simulink model "AutonomousControl"  (R2015a)
settings: Solver=ode45  StartTime=0.0  StopTime=inf  FixedStep=0.01  RelTol=1e-3
libraries: simulink x11, dspindex x8, dspnetwork x3, aerolibconvert2 x1, IMU_Library x1, GPS_Library x1, realtime_pacer_lib x1, etargetslib x1
(part 1 of 2)
settings Model: xpc_rtwmakecfg_data=_xpcnblib__xpcetherlib__xpcether8255xlib__xpcetherGbElib__xpciplib_  ParamWorkspaceSource=ReferencedWorkspace  CovSFcnEnable=off  Creator=abdkadma  LastModifiedBy=theth
settings OptimizationCC: InlineParams=on  InlineInvariantSignals=on  EnhancedBackFolding=on  ExpressionDepthLimit=2147483647  EfficientFloat2IntCast=on  SimCompilerOptimization=on
settings DebuggingCC: UnderspecifiedInitializationDetection=Classic  MergeDetectMultiDrivingBlocksExec=none  SolverPrmCheckMsg=warning  StateNameClashWarn=warning
settings RTWCC: RTWCompilerOptimization=on  CheckMdlBeforeBuild=Warning
settings GRTTargetCC: MatFileLogging=off  SupportNonFinite=off

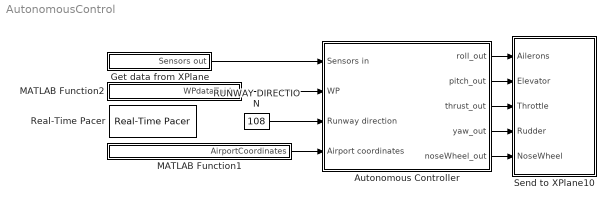
== system AutonomousControl ==
  "Autonomous Controller " : Subsystem
  Get data from XPlane : Subsystem  Description=|  TreatAsAtomicUnit=on  mask(Get Data from Xplane10){remoteURL='127.0.0.1', localPort=49005, sampletime=0.02}
      | Done by: Mohamed Abdelkader
      | Contact for updates: mohamedashraf123@gmail.com
      mask prompts: remoteURL "Remote IP address ('0.0.0.0' to accept all):(default='127.0.0.1')"; localPort "Local IP port: that Xplane10 sends to (default=49005)"; sampletime "Sampling time (seconds), how frequenlty to capture data from Xplane. Don't set to low as it might not be able to capture the smaples from Xplane. Default is 0.02 assuming the UDP rate in Xplane is set to 50 sample per second"
      mask help:
      | Get Data from X-Plane10
      | * make sure you configure the right port
      | and the right IP address
      mask TypeOptions remoteURL: UDP Receive1/remoteURL
      mask TypeOptions localPort: UDP Receive1/localPort
      mask TypeOptions sampletime: UDP Receive1/sampletime
  MATLAB Function1 : MATLAB Function  TreatAsAtomicUnit=on
  MATLAB Function2 : MATLAB Function  TreatAsAtomicUnit=on
  RUNWAY DIRECTION : Constant  Value=108
  Real-Time Pacer : realtime_pacer_lib/Real-Time Pacer  simTimePerRealTime=1
  Send to XPlane10 : Subsystem  Description=|  mask(Send Commands to X-Plane 10){remoteURL='127.0.0.1', remotePort=49000}
      | Done by: Mohamed Abdelkader
      | Contact for updates: mohamedashraf123@gmail.com
      mask prompts: remoteURL "Remote IP address (default='127.0.0.1'): X-Plane10 IP"; remotePort "Remote IP port:X-Plane10 port(default=49000)"
      mask help:
      | Sends Control Surfaces Commands to Xplane10
      | Throttle in [0,1]
      | Elevator, Ailerons, rudder, nosewheel in [-1,1]
      mask TypeOptions remoteURL: UDP Send/remoteURL
      mask TypeOptions remotePort: UDP Send/remotePort
  wires:
  "Autonomous Controller "/1(roll_out) -> Send to XPlane10/1(Ailerons)
  "Autonomous Controller "/2(pitch_out) -> Send to XPlane10/2(Elevator)
  "Autonomous Controller "/3(thrust_out) -> Send to XPlane10/3(Throttle)
  "Autonomous Controller "/4(yaw_out) -> Send to XPlane10/4(Rudder)
  "Autonomous Controller "/5(noseWheel_out) -> Send to XPlane10/5(NoseWheel)
  Get data from XPlane/1(Sensors out) -> "Autonomous Controller "/1(Sensors in)
  RUNWAY DIRECTION/1 -> "Autonomous Controller "/3(Runway direction)
  MATLAB Function1/1(AirportCoordinates) -> "Autonomous Controller "/4(Airport coordinates)
  MATLAB Function2/1(WPdataTable) -> "Autonomous Controller "/2(WP)

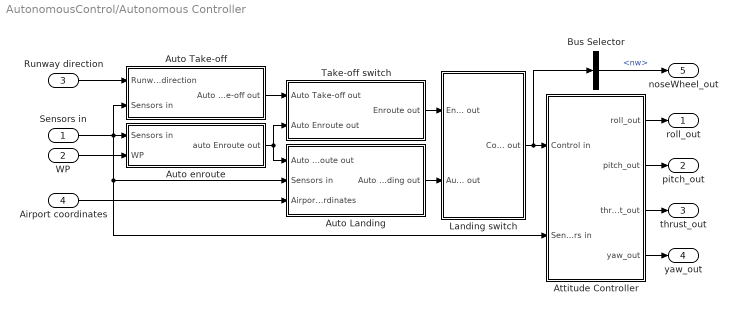
== system AutonomousControl/Autonomous Controller  ==
  Sensors in : Inport
  WP : Inport  Port=2
  Runway direction : Inport  Port=3
  Airport coordinates : Inport  Port=4
  Attitude Controller : Subsystem
  Auto Landing : Subsystem
  Auto Take-off : Subsystem
  Auto enroute : Subsystem
  Bus Selector : BusSelector  OutputSignals=nw
  Landing switch : Subsystem
  Take-off switch : Subsystem
  roll_out : Outport
  pitch_out : Outport  Port=2
  thrust_out : Outport  Port=3
  yaw_out : Outport  Port=4
  noseWheel_out : Outport  Port=5
  wires:
  Take-off switch/1(Enroute out) -> Landing switch/1(Enroute out)
  Auto Landing/1(Auto Landing out) -> Landing switch/2(Auto landing out)
  Auto enroute/1(auto Enroute out) -> Take-off switch/2(Auto Enroute out), Auto Landing/1(Auto Enroute out)
  Attitude Controller/4(yaw_out) -> yaw_out/1
  Attitude Controller/1(roll_out) -> roll_out/1
  Attitude Controller/3(thrust_out) -> thrust_out/1
  Auto Take-off/1(Auto Take-off out) -> Take-off switch/1(Auto Take-off out)
  Sensors in/1 -> Auto Take-off/2(Sensors in), Auto Landing/2(Sensors in), Attitude Controller/2(Sensors in), Auto enroute/1(Sensors in)
  Runway direction/1 -> Auto Take-off/1(Runway direction)
  Landing switch/1(Control out) -> Bus Selector/1, Attitude Controller/1(Control in)
  Bus Selector/1 -> noseWheel_out/1  "<nw>"
  Attitude Controller/2(pitch_out) -> pitch_out/1
  Airport coordinates/1 -> Auto Landing/3(Airport coordinates)
  WP/1 -> Auto enroute/2(WP)

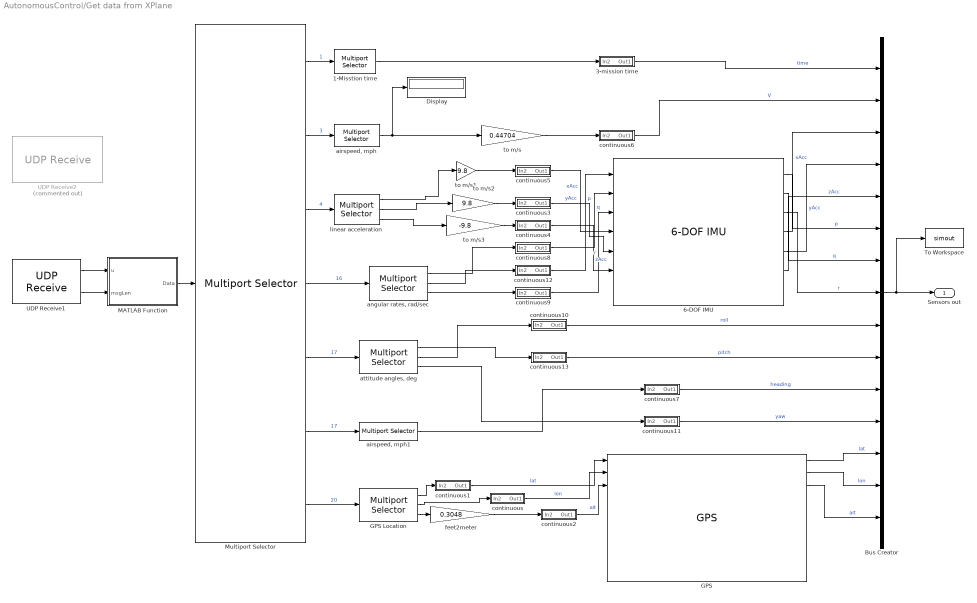
== system AutonomousControl/Get data from XPlane ==
  1-Misstion time : dspindex/Multiport Selector  rowsOrCols=Columns  idxCellArray={3}  idxErrMode=Clip Index
  3-mission time : Subsystem
  6-DOF IMU : IMU_Library/6-DOF IMU  lpf_filt_freq_hz_ix=20 Hz  gyro_scale_ix=+/- 500 deg/sec  accel_scale_ix=+/- 8g  SampleTime=0.02  lpf_filt_freq_hz=5 Hz  gyro_scale=+/- 250 deg/sec  accel_scale=+/- 2g
  Bus Creator : BusCreator  Inputs='time','V','xAcc','yAcc','zAcc','p','q','r','roll','pitch','heading','yaw','lat','lon','alt'
  Display : Display
  GPS : GPS_Library/GPS
  GPS Location : dspindex/Multiport Selector  rowsOrCols=Columns  idxCellArray={1,2,3}  idxErrMode=Clip Index
  MATLAB Function : MATLAB Function  TreatAsAtomicUnit=on
  Multiport Selector : dspindex/Multiport Selector  rowsOrCols=Rows  idxCellArray={1,3,4,16,17,18,20}  idxErrMode=Clip Index
  To Workspace : ToWorkspace  VariableName=simout  SampleTime=-1
      settings: Save2DSignal=2-D array (concatenate along first dimension)
  UDP Receive1 : dspnetwork/UDP Receive  localURL='0.0.0.0'  localPort=localPort  remoteURL=remoteURL  remotePort=-1  recvBufferSize=8192  dims=365*20  signalDatatype=uint8  isVarSize=off  showBlockingTime=off  blockingTime=0  sampletime=sampletime
  UDP Receive2 : dspnetwork/UDP Receive  Commented=on  localURL='0.0.0.0'  localPort=localPort  remoteURL=remoteURL  remotePort=-1  recvBufferSize=8192  dims=365  signalDatatype=uint8  isVarSize=off  showBlockingTime=on  blockingTime=0.01  sampletime=0.01  blockPlatform=LINUX
  "airspeed, mph" : dspindex/Multiport Selector  rowsOrCols=Columns  idxCellArray={6}  idxErrMode=Clip Index
  "airspeed, mph1" : dspindex/Multiport Selector  rowsOrCols=Columns  idxCellArray={3}  idxErrMode=Clip Index
  "angular rates, rad/sec" : dspindex/Multiport Selector  rowsOrCols=Columns  idxCellArray={1,2,3}  idxErrMode=Clip Index
  "attitude angles, deg" : dspindex/Multiport Selector  rowsOrCols=Columns  idxCellArray={1,2,3}  idxErrMode=Clip Index
  continuous : Subsystem
  continuous1 : Subsystem
  continuous10 : Subsystem
  continuous11 : Subsystem
  continuous12 : Subsystem
  continuous13 : Subsystem
  continuous2 : Subsystem
  continuous3 : Subsystem
  continuous4 : Subsystem
  continuous5 : Subsystem
  continuous6 : Subsystem
  continuous7 : Subsystem
  continuous8 : Subsystem
  continuous9 : Subsystem
  feet2meter : Gain  Gain=0.3048
  linear acceleration : dspindex/Multiport Selector  rowsOrCols=Columns  idxCellArray={6,7,5}  idxErrMode=Clip Index
  to m/s : Gain  Gain=0.44704
  to m/s1 : Gain  Gain=9.8
  to m/s2 : Gain  Gain=9.8
  to m/s3 : Gain  Gain=-9.8
  Sensors out : Outport
  wires:
  "attitude angles, deg"/3 -> continuous11/1(In2)
  "angular rates, rad/sec"/3 -> continuous9/1(In2)
  MATLAB Function/1(Data) -> Multiport Selector/1
  linear acceleration/2 -> to m/s2/1
  to m/s2/1 -> continuous3/1(In2)
  to m/s1/1 -> continuous5/1(In2)
  "attitude angles, deg"/1 -> continuous13/1(In2)
  "attitude angles, deg"/2 -> continuous10/1(In2)
  to m/s/1 -> continuous6/1(In2)
  "airspeed, mph"/1 -> Display/1, to m/s/1
  linear acceleration/1 -> to m/s1/1
  "angular rates, rad/sec"/1 -> continuous8/1(In2)
  linear acceleration/3 -> to m/s3/1
  "angular rates, rad/sec"/2 -> continuous12/1(In2)
  "airspeed, mph1"/1 -> continuous7/1(In2)
  to m/s3/1 -> continuous4/1(In2)
  feet2meter/1 -> continuous2/1(In2)
  UDP Receive1/1 -> MATLAB Function/1(u)
  UDP Receive1/2 -> MATLAB Function/2(msgLen)
  GPS Location/3 -> feet2meter/1
  GPS Location/1 -> continuous1/1(In2)
  continuous6/1(Out1) -> Bus Creator/2  "V"
  continuous7/1(Out1) -> Bus Creator/11  "heading"
  continuous10/1(Out1) -> Bus Creator/9  "roll"
  continuous11/1(Out1) -> Bus Creator/12  "yaw"
  continuous13/1(Out1) -> Bus Creator/10  "pitch"
  Bus Creator/1 -> To Workspace/1, Sensors out/1
  Multiport Selector/4 -> "angular rates, rad/sec"/1  "16"
  Multiport Selector/5 -> "attitude angles, deg"/1  "17"
  Multiport Selector/6 -> "airspeed, mph1"/1  "17"
  Multiport Selector/7 -> GPS Location/1  "20"
  1-Misstion time/1 -> 3-mission time/1(In2)
  3-mission time/1(Out1) -> Bus Creator/1  "time"
  Multiport Selector/1 -> 1-Misstion time/1  "1"
  Multiport Selector/2 -> "airspeed, mph"/1  "3"
  Multiport Selector/3 -> linear acceleration/1  "4"
  continuous5/1(Out1) -> 6-DOF IMU/4  "xAcc"
  6-DOF IMU/4 -> Bus Creator/3  "xAcc"
  continuous3/1(Out1) -> 6-DOF IMU/5  "yAcc"
  6-DOF IMU/5 -> Bus Creator/4  "yAcc"
  continuous4/1(Out1) -> 6-DOF IMU/6  "zAcc"
  6-DOF IMU/6 -> Bus Creator/5  "zAcc"
  continuous12/1(Out1) -> 6-DOF IMU/1  "p"
  continuous8/1(Out1) -> 6-DOF IMU/2  "q"
  continuous9/1(Out1) -> 6-DOF IMU/3  "r"
  6-DOF IMU/1 -> Bus Creator/6  "p"
  6-DOF IMU/2 -> Bus Creator/7  "q"
  6-DOF IMU/3 -> Bus Creator/8  "r"
  continuous1/1(Out1) -> GPS/1  "lat"
  GPS/1 -> Bus Creator/13  "lat"
  continuous/1(Out1) -> GPS/2  "lon"
  GPS/2 -> Bus Creator/14  "lon"
  continuous2/1(Out1) -> GPS/3  "alt"
  GPS/3 -> Bus Creator/15  "alt"
  GPS Location/2 -> continuous/1(In2)

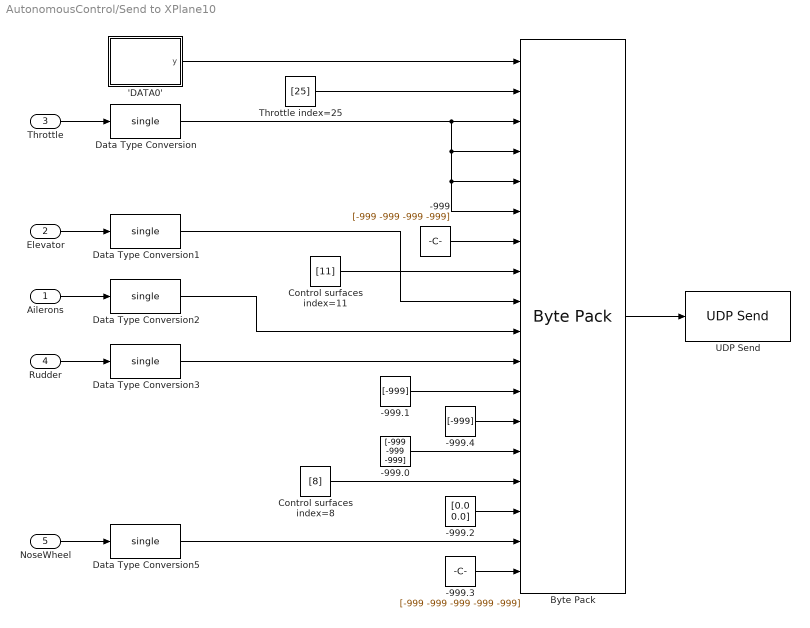
== system AutonomousControl/Send to XPlane10 ==
  Ailerons : Inport
  Elevator : Inport  Port=2
  Throttle : Inport  Port=3
  Rudder : Inport  Port=4
  NoseWheel : Inport  Port=5
  'DATA0' : MATLAB Function  TreatAsAtomicUnit=on
  -999 : Constant  Value=[-999 -999 -999 -999]  OutDataTypeStr=int32  SampleTime=-1
  -999.0 : Constant  Value=[-999 -999 -999]  OutDataTypeStr=int32  SampleTime=-1
  -999.1 : Constant  Value=[-999]  OutDataTypeStr=int32  SampleTime=-1
  -999.2 : Constant  Value=[0.0 0.0]  OutDataTypeStr=single  SampleTime=-1
  -999.3 : Constant  Value=[-999 -999 -999 -999 -999]  OutDataTypeStr=int32  SampleTime=-1
  -999.4 : Constant  Value=[-999]  OutDataTypeStr=single  SampleTime=-1
  Byte Pack : etargetslib/Byte Pack  datatypes={'uint8','uint32','single','single','single','single','int32','uint32','single','single','single','int32','single','int32','uint32','single','single','int32'}  byteAlign=1
  Control surfaces index=11 : Constant  Value=[11]  OutDataTypeStr=uint32  SampleTime=-1
  Control surfaces index=8 : Constant  Value=[8]  OutDataTypeStr=uint32  SampleTime=-1
  Data Type Conversion : DataTypeConversion  OutMin=[0]  OutMax=[1.0]  OutDataTypeStr=single
  Data Type Conversion{1..3,5} (4 alike) : DataTypeConversion  OutMin=[-1.0]  OutMax=[1.0]  OutDataTypeStr=single
  Throttle index=25 : Constant  Value=[25]  OutDataTypeStr=uint32  SampleTime=-1
  UDP Send : dspnetwork/UDP Send  remoteURL=remoteURL  remotePort=remotePort  localURL='0.0.0.0'  localPortSource=Automatically determine  localPort=-1  sampletime=-1  separateLengthPort=0
  wires:
  Ailerons/1 -> Data Type Conversion2/1
  Control surfaces index=11/1 -> Byte Pack/8
  Throttle/1 -> Data Type Conversion/1
  Data Type Conversion1/1 -> Byte Pack/9
  'DATA0'/1(y) -> Byte Pack/1
  Throttle index=25/1 -> Byte Pack/2
  Byte Pack/1 -> UDP Send/1
  -999/1 -> Byte Pack/7
  Data Type Conversion2/1 -> Byte Pack/10
  Data Type Conversion3/1 -> Byte Pack/11
  Rudder/1 -> Data Type Conversion3/1
  -999.0/1 -> Byte Pack/14
  Elevator/1 -> Data Type Conversion1/1
  Data Type Conversion/1 -> Byte Pack/3, Byte Pack/4, Byte Pack/6, Byte Pack/5
  -999.1/1 -> Byte Pack/12
  Control surfaces index=8/1 -> Byte Pack/15
  -999.2/1 -> Byte Pack/16
  Data Type Conversion5/1 -> Byte Pack/17
  NoseWheel/1 -> Data Type Conversion5/1
  -999.3/1 -> Byte Pack/18
  -999.4/1 -> Byte Pack/13

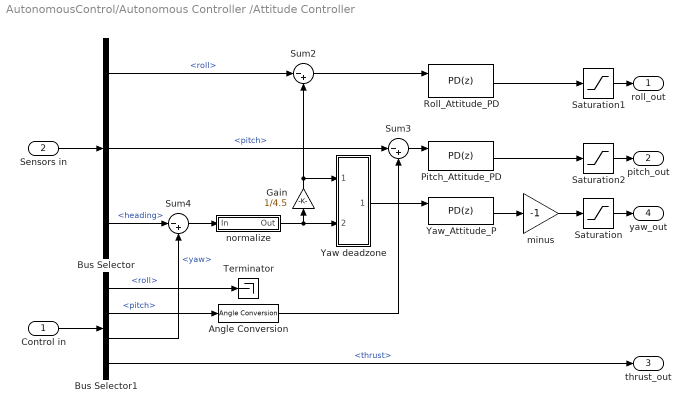
== system AutonomousControl/Autonomous Controller /Attitude Controller ==
  Control in : Inport
  Sensors in : Inport  Port=2
  Angle Conversion : aerolibconvert2/Angle Conversion  IU=rad  OU=deg
  Bus Selector : BusSelector  OutputSignals=roll,pitch,heading
  Bus Selector1 : BusSelector  OutputSignals=roll,pitch,yaw,thrust
  Gain : Gain  Gain=1/4.5
  Pitch_Attitude_PD : simulink/Continuous/PID Controller  Controller=PD  TimeDomain=Discrete-time  SampleTime=0.02  IntegratorMethod=Forward Euler  FilterMethod=Forward Euler  Form=Parallel  UseFilter=off  ControllerParametersSource=internal  P=1*pi/180  I=0  D=0.04*pi/180  N=20  InitialConditionSource=internal  InitialConditionForIntegrator=0  InitialConditionForFilter=0  ExternalReset=either  LimitOutput=on  UpperSaturationLimit=1  LowerSaturationLimit=-1  LinearizeAsGain=on  AntiWindupMode=none  Kb=1  TrackingMode=off  Kt=1  PParamMin=[]  PParamMax=[]  IParamMin=[]  IParamMax=[]  DParamMin=[]  DParamMax=[]  NParamMin=[]  NParamMax=[]  KbParamMin=[]  KbParamMax=[]  KtParamMin=[]  KtParamMax=[]  POutMin=[]  POutMax=[]  IOutMin=[]  IOutMax=[]  DOutMin=[]  DOutMax=[]  NOutMin=[]  NOutMax=[]  KbOutMin=[]  KbOutMax=[]  KtOutMin=[]  KtOutMax=[]  IntegratorOutMin=[]  IntegratorOutMax=[]  FilterOutMin=[]  FilterOutMax=[]  SumOutMin=[]  SumOutMax=[]  SumI1OutMin=[]  SumI1OutMax=[]  SumI2OutMin=[]  SumI2OutMax=[]  SumI3OutMin=[]  SumI3OutMax=[]  SumDOutMin=[]  SumDOutMax=[]  SaturationOutMin=[]  SaturationOutMax=[]  IntegratorContinuousStateAttributes=''  IntegratorStateMustResolveToSignalObject=off  IntegratorRTWStateStorageClass=Auto  FilterContinuousStateAttributes=''  FilterStateMustResolveToSignalObject=off  FilterRTWStateStorageClass=Auto  DifferentiatorICPrevScaledInput=0  DifferentiatorOutMin=[]  DifferentiatorOutMax=[]
  Roll_Attitude_PD : simulink/Continuous/PID Controller  Controller=PD  TimeDomain=Discrete-time  SampleTime=0.02  IntegratorMethod=Forward Euler  FilterMethod=Forward Euler  Form=Parallel  UseFilter=off  ControllerParametersSource=internal  P=pi/180/4  I=0  D=0.0008*pi/180/4  N=20  InitialConditionSource=internal  InitialConditionForIntegrator=0  InitialConditionForFilter=0  ExternalReset=either  LimitOutput=on  UpperSaturationLimit=1  LowerSaturationLimit=-1  LinearizeAsGain=on  AntiWindupMode=none  Kb=1  TrackingMode=off  Kt=1  PParamMin=[]  PParamMax=[]  IParamMin=[]  IParamMax=[]  DParamMin=[]  DParamMax=[]  NParamMin=[]  NParamMax=[]  KbParamMin=[]  KbParamMax=[]  KtParamMin=[]  KtParamMax=[]  POutMin=[]  POutMax=[]  IOutMin=[]  IOutMax=[]  DOutMin=[]  DOutMax=[]  NOutMin=[]  NOutMax=[]  KbOutMin=[]  KbOutMax=[]  KtOutMin=[]  KtOutMax=[]  IntegratorOutMin=[]  IntegratorOutMax=[]  FilterOutMin=[]  FilterOutMax=[]  SumOutMin=[]  SumOutMax=[]  SumI1OutMin=[]  SumI1OutMax=[]  SumI2OutMin=[]  SumI2OutMax=[]  SumI3OutMin=[]  SumI3OutMax=[]  SumDOutMin=[]  SumDOutMax=[]  SaturationOutMin=[]  SaturationOutMax=[]  IntegratorContinuousStateAttributes=''  IntegratorStateMustResolveToSignalObject=off  IntegratorRTWStateStorageClass=Auto  FilterContinuousStateAttributes=''  FilterStateMustResolveToSignalObject=off  FilterRTWStateStorageClass=Auto  DifferentiatorICPrevScaledInput=0  DifferentiatorOutMin=[]  DifferentiatorOutMax=[]
  Saturation : Saturate  UpperLimit=1  LowerLimit=-1
  Saturation1 : Saturate  UpperLimit=0.05  LowerLimit=-0.05
  Saturation2 : Saturate  UpperLimit=1  LowerLimit=-1
  Sum2 : Sum  Inputs=|-+
  Sum3 : Sum  Inputs=|-+
  Sum4 : Sum  Inputs=|-+
  Terminator : Terminator
  Yaw deadzone : Subsystem
  Yaw_Attitude_P : simulink/Continuous/PID Controller  Controller=PD  TimeDomain=Discrete-time  SampleTime=0.02  IntegratorMethod=Forward Euler  FilterMethod=Forward Euler  Form=Parallel  UseFilter=off  ControllerParametersSource=internal  P=6*pi/180  I=0  D=6*0.000034  N=100  InitialConditionSource=internal  InitialConditionForIntegrator=0  InitialConditionForFilter=0  ExternalReset=either  LimitOutput=on  UpperSaturationLimit=1  LowerSaturationLimit=-1  LinearizeAsGain=on  AntiWindupMode=none  Kb=1  TrackingMode=off  Kt=1  PParamMin=[]  PParamMax=[]  IParamMin=[]  IParamMax=[]  DParamMin=[]  DParamMax=[]  NParamMin=[]  NParamMax=[]  KbParamMin=[]  KbParamMax=[]  KtParamMin=[]  KtParamMax=[]  POutMin=[]  POutMax=[]  IOutMin=[]  IOutMax=[]  DOutMin=[]  DOutMax=[]  NOutMin=[]  NOutMax=[]  KbOutMin=[]  KbOutMax=[]  KtOutMin=[]  KtOutMax=[]  IntegratorOutMin=[]  IntegratorOutMax=[]  FilterOutMin=[]  FilterOutMax=[]  SumOutMin=[]  SumOutMax=[]  SumI1OutMin=[]  SumI1OutMax=[]  SumI2OutMin=[]  SumI2OutMax=[]  SumI3OutMin=[]  SumI3OutMax=[]  SumDOutMin=[]  SumDOutMax=[]  SaturationOutMin=[]  SaturationOutMax=[]  IntegratorContinuousStateAttributes=''  IntegratorStateMustResolveToSignalObject=off  IntegratorRTWStateStorageClass=Auto  FilterContinuousStateAttributes=''  FilterStateMustResolveToSignalObject=off  FilterRTWStateStorageClass=Auto  DifferentiatorICPrevScaledInput=0  DifferentiatorOutMin=[]  DifferentiatorOutMax=[]
  minus : Gain  Gain=-1
  normalize : Subsystem
  roll_out : Outport
  pitch_out : Outport  Port=2
  thrust_out : Outport  Port=3
  yaw_out : Outport  Port=4
  wires:
  Sum2/1 -> Roll_Attitude_PD/1
  Sum3/1 -> Pitch_Attitude_PD/1
  Bus Selector/1 -> Sum2/1  "<roll>"
  Bus Selector/2 -> Sum3/1  "<pitch>"
  minus/1 -> Saturation/1
  Bus Selector/3 -> Sum4/1  "<heading>"
  Sum4/1 -> normalize/1(In)
  Sensors in/1 -> Bus Selector/1
  Control in/1 -> Bus Selector1/1
  Bus Selector1/2 -> Angle Conversion/1  "<pitch>"
  Bus Selector1/4 -> thrust_out/1  "<thrust>"
  Bus Selector1/3 -> Sum4/2  "<yaw>"
  Saturation1/1 -> roll_out/1
  Saturation2/1 -> pitch_out/1
  Yaw_Attitude_P/1 -> minus/1
  Pitch_Attitude_PD/1 -> Saturation2/1
  Roll_Attitude_PD/1 -> Saturation1/1
  Saturation/1 -> yaw_out/1
  Gain/1 -> Sum2/2, Yaw deadzone/1(Roll)
  Angle Conversion/1 -> Sum3/2
  normalize/1(Out) -> Gain/1, Yaw deadzone/2(in)
  Yaw deadzone/1(out) -> Yaw_Attitude_P/1
  Bus Selector1/1 -> Terminator/1  "<roll>"

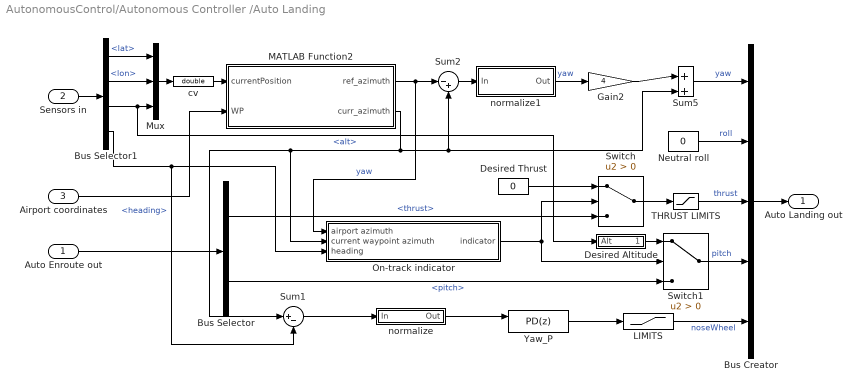
== system AutonomousControl/Autonomous Controller /Auto Landing ==
  Auto Enroute out : Inport
  Sensors in : Inport  Port=2
  Airport coordinates : Inport  Port=3
  Bus Creator : BusCreator  Inputs='yaw','roll','thrust','pitch','noseWheel'
  Bus Selector : BusSelector  OutputSignals=thrust,pitch
  Bus Selector1 : BusSelector  OutputSignals=lat,lon,alt,heading
  Desired Altitude : Subsystem
  Desired Thrust : Constant  Value=0  OutDataTypeStr=single
  Gain2 : Gain  Gain=4
  LIMITS : Saturate
  MATLAB Function2 : MATLAB Function  TreatAsAtomicUnit=on
  Mux : Mux  Inputs=3
  Neutral roll : Constant  Value=0  OutDataTypeStr=single
  On-track indicator : Subsystem
  Sum1 : Sum  Inputs=|+-
  Sum2 : Sum  Inputs=|-+
  Sum5 : Sum  Inputs=|++
  Switch : Switch  Criteria=u2 > Threshold
  Switch1 : Switch  Criteria=u2 > Threshold
  THRUST LIMITS : Saturate  UpperLimit=1  LowerLimit=0
  Yaw_P : simulink/Continuous/PID Controller  Controller=PD  TimeDomain=Discrete-time  SampleTime=0.05  IntegratorMethod=Forward Euler  FilterMethod=Forward Euler  Form=Parallel  UseFilter=off  ControllerParametersSource=internal  P=0.016  I=0  D=0.0024  N=100  InitialConditionSource=internal  InitialConditionForIntegrator=0  InitialConditionForFilter=0  ExternalReset=either  LimitOutput=on  UpperSaturationLimit=1  LowerSaturationLimit=-1  LinearizeAsGain=on  AntiWindupMode=none  Kb=1  TrackingMode=off  Kt=1  PParamMin=[]  PParamMax=[]  IParamMin=[]  IParamMax=[]  DParamMin=[]  DParamMax=[]  NParamMin=[]  NParamMax=[]  KbParamMin=[]  KbParamMax=[]  KtParamMin=[]  KtParamMax=[]  POutMin=[]  POutMax=[]  IOutMin=[]  IOutMax=[]  DOutMin=[]  DOutMax=[]  NOutMin=[]  NOutMax=[]  KbOutMin=[]  KbOutMax=[]  KtOutMin=[]  KtOutMax=[]  IntegratorOutMin=[]  IntegratorOutMax=[]  FilterOutMin=[]  FilterOutMax=[]  SumOutMin=[]  SumOutMax=[]  SumI1OutMin=[]  SumI1OutMax=[]  SumI2OutMin=[]  SumI2OutMax=[]  SumI3OutMin=[]  SumI3OutMax=[]  SumDOutMin=[]  SumDOutMax=[]  SaturationOutMin=[]  SaturationOutMax=[]  IntegratorContinuousStateAttributes=''  IntegratorStateMustResolveToSignalObject=off  IntegratorRTWStateStorageClass=Auto  FilterContinuousStateAttributes=''  FilterStateMustResolveToSignalObject=off  FilterRTWStateStorageClass=Auto  DifferentiatorICPrevScaledInput=0  DifferentiatorOutMin=[]  DifferentiatorOutMax=[]
  cv : DataTypeConversion  OutDataTypeStr=double
  normalize : Subsystem
  normalize1 : Subsystem
  Auto Landing out : Outport
  wires:
  THRUST LIMITS/1 -> Bus Creator/3  "thrust"
  Airport coordinates/1 -> MATLAB Function2/2(WP)
  MATLAB Function2/2(curr_azimuth) -> Sum1/1, On-track indicator/2(current waypoint azimuth), Sum5/2, Sum2/2
  LIMITS/1 -> Bus Creator/5  "noseWheel"
  MATLAB Function2/1(ref_azimuth) -> Sum2/1, On-track indicator/1(airport azimuth)  "yaw"
  normalize/1(Out) -> Yaw_P/1
  Auto Enroute out/1 -> Bus Selector/1
  Bus Selector/1 -> Switch/3  "<thrust>"
  Neutral roll/1 -> Bus Creator/2  "roll"
  Sum1/1 -> normalize/1(In)
  Bus Creator/1 -> Auto Landing out/1
  Sensors in/1 -> Bus Selector1/1
  Bus Selector1/1 -> Mux/1  "<lat>"
  Bus Selector1/2 -> Mux/2  "<lon>"
  Bus Selector1/3 -> Desired Altitude/1(Alt), Mux/3  "<alt>"
  Sum2/1 -> normalize1/1(In)
  Bus Selector1/4 -> Sum1/2, On-track indicator/3(heading)  "<heading>"
  Desired Thrust/1 -> Switch/1
  Bus Selector/2 -> Switch1/3  "<pitch>"
  Switch/1 -> THRUST LIMITS/1
  Switch1/1 -> Bus Creator/4  "pitch"
  normalize1/1(Out) -> Gain2/1  "yaw"
  Sum5/1 -> Bus Creator/1  "yaw"
  On-track indicator/1(indicator) -> Switch1/2, Switch/2
  Gain2/1 -> Sum5/1
  Mux/1 -> cv/1
  cv/1 -> MATLAB Function2/1(currentPosition)
  Yaw_P/1 -> LIMITS/1
  Desired Altitude/1(pitch) -> Switch1/1

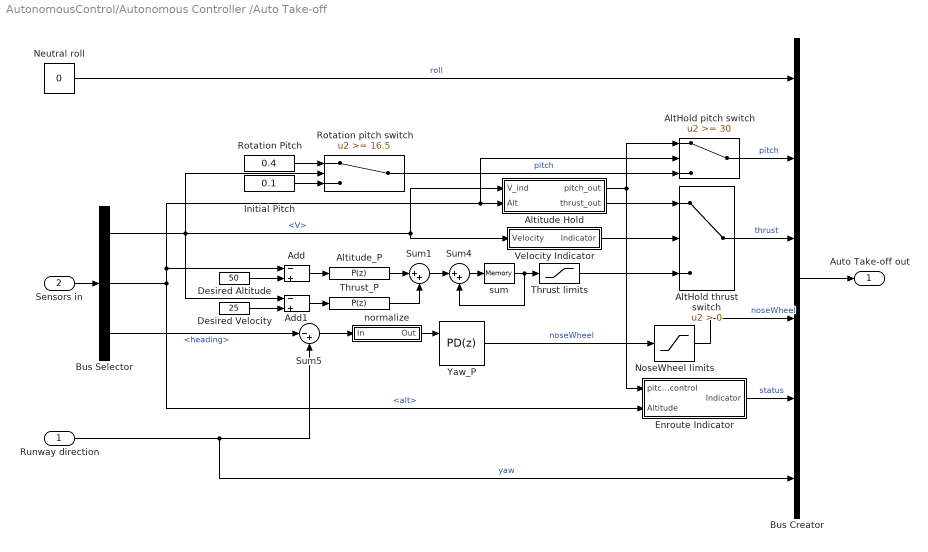
== system AutonomousControl/Autonomous Controller /Auto Take-off ==
  Runway direction : Inport
  Sensors in : Inport  Port=2
  Add : Sum  Inputs=-+
  Add1 : Sum  Inputs=-+
  AltHold pitch switch : Switch  Threshold=30
  AltHold thrust switch : Switch  Criteria=u2 > Threshold
  Altitude Hold : Subsystem
  Altitude_P : simulink/Continuous/PID Controller  Controller=P  TimeDomain=Discrete-time  SampleTime=-1  IntegratorMethod=Forward Euler  FilterMethod=Forward Euler  Form=Parallel  UseFilter=on  ControllerParametersSource=internal  P=0.1  I=0  D=0.01  N=20  InitialConditionSource=internal  InitialConditionForIntegrator=0  InitialConditionForFilter=0  ExternalReset=either  LimitOutput=on  UpperSaturationLimit=1  LowerSaturationLimit=-1  LinearizeAsGain=on  AntiWindupMode=none  Kb=1  TrackingMode=off  Kt=1  PParamMin=[]  PParamMax=[]  IParamMin=[]  IParamMax=[]  DParamMin=[]  DParamMax=[]  NParamMin=[]  NParamMax=[]  KbParamMin=[]  KbParamMax=[]  KtParamMin=[]  KtParamMax=[]  POutMin=[]  POutMax=[]  IOutMin=[]  IOutMax=[]  DOutMin=[]  DOutMax=[]  NOutMin=[]  NOutMax=[]  KbOutMin=[]  KbOutMax=[]  KtOutMin=[]  KtOutMax=[]  IntegratorOutMin=[]  IntegratorOutMax=[]  FilterOutMin=[]  FilterOutMax=[]  SumOutMin=[]  SumOutMax=[]  SumI1OutMin=[]  SumI1OutMax=[]  SumI2OutMin=[]  SumI2OutMax=[]  SumI3OutMin=[]  SumI3OutMax=[]  SumDOutMin=[]  SumDOutMax=[]  SaturationOutMin=[]  SaturationOutMax=[]  IntegratorContinuousStateAttributes=''  IntegratorStateMustResolveToSignalObject=off  IntegratorRTWStateStorageClass=Auto  FilterContinuousStateAttributes=''  FilterStateMustResolveToSignalObject=off  FilterRTWStateStorageClass=Auto  DifferentiatorICPrevScaledInput=0  DifferentiatorOutMin=[]  DifferentiatorOutMax=[]
  Bus Creator : BusCreator  Inputs='roll','pitch','thrust','noseWheel','status','yaw'
  Bus Selector : BusSelector  OutputSignals=V,alt,heading
  Desired Altitude : Constant  Value=50  OutDataTypeStr=single
  Desired Velocity : Constant  Value=25  OutDataTypeStr=single
  Enroute Indicator : Subsystem
  Initial Pitch : Constant  Value=0.1  OutDataTypeStr=single
  Neutral roll : Constant  Value=0  OutDataTypeStr=single
  NoseWheel limits : Saturate
  Rotation Pitch : Constant  Value=0.4  OutDataTypeStr=single
  Rotation pitch switch : Switch  Threshold=16.5
  Sum1 : Sum  Inputs=|++
  Sum4 : Sum  Inputs=|++
  Sum5 : Sum  Inputs=|-+
  Thrust limits : Saturate  UpperLimit=1  LowerLimit=0
  Thrust_P : simulink/Continuous/PID Controller  Controller=P  TimeDomain=Discrete-time  SampleTime=-1  IntegratorMethod=Forward Euler  FilterMethod=Forward Euler  Form=Parallel  UseFilter=on  ControllerParametersSource=internal  P=0.1  I=0  D=0.01  N=20  InitialConditionSource=internal  InitialConditionForIntegrator=0  InitialConditionForFilter=0  ExternalReset=either  LimitOutput=on  UpperSaturationLimit=1  LowerSaturationLimit=-1  LinearizeAsGain=on  AntiWindupMode=none  Kb=1  TrackingMode=off  Kt=1  PParamMin=[]  PParamMax=[]  IParamMin=[]  IParamMax=[]  DParamMin=[]  DParamMax=[]  NParamMin=[]  NParamMax=[]  KbParamMin=[]  KbParamMax=[]  KtParamMin=[]  KtParamMax=[]  POutMin=[]  POutMax=[]  IOutMin=[]  IOutMax=[]  DOutMin=[]  DOutMax=[]  NOutMin=[]  NOutMax=[]  KbOutMin=[]  KbOutMax=[]  KtOutMin=[]  KtOutMax=[]  IntegratorOutMin=[]  IntegratorOutMax=[]  FilterOutMin=[]  FilterOutMax=[]  SumOutMin=[]  SumOutMax=[]  SumI1OutMin=[]  SumI1OutMax=[]  SumI2OutMin=[]  SumI2OutMax=[]  SumI3OutMin=[]  SumI3OutMax=[]  SumDOutMin=[]  SumDOutMax=[]  SaturationOutMin=[]  SaturationOutMax=[]  IntegratorContinuousStateAttributes=''  IntegratorStateMustResolveToSignalObject=off  IntegratorRTWStateStorageClass=Auto  FilterContinuousStateAttributes=''  FilterStateMustResolveToSignalObject=off  FilterRTWStateStorageClass=Auto  DifferentiatorICPrevScaledInput=0  DifferentiatorOutMin=[]  DifferentiatorOutMax=[]
  Velocity Indicator : Subsystem
  Yaw_P : simulink/Continuous/PID Controller  Controller=PD  TimeDomain=Discrete-time  SampleTime=0.02  IntegratorMethod=Forward Euler  FilterMethod=Forward Euler  Form=Parallel  UseFilter=off  ControllerParametersSource=internal  P=0.012  I=0  D=0.0024  N=100  InitialConditionSource=internal  InitialConditionForIntegrator=0  InitialConditionForFilter=0  ExternalReset=either  LimitOutput=on  UpperSaturationLimit=1  LowerSaturationLimit=-1  LinearizeAsGain=on  AntiWindupMode=none  Kb=1  TrackingMode=off  Kt=1  PParamMin=[]  PParamMax=[]  IParamMin=[]  IParamMax=[]  DParamMin=[]  DParamMax=[]  NParamMin=[]  NParamMax=[]  KbParamMin=[]  KbParamMax=[]  KtParamMin=[]  KtParamMax=[]  POutMin=[]  POutMax=[]  IOutMin=[]  IOutMax=[]  DOutMin=[]  DOutMax=[]  NOutMin=[]  NOutMax=[]  KbOutMin=[]  KbOutMax=[]  KtOutMin=[]  KtOutMax=[]  IntegratorOutMin=[]  IntegratorOutMax=[]  FilterOutMin=[]  FilterOutMax=[]  SumOutMin=[]  SumOutMax=[]  SumI1OutMin=[]  SumI1OutMax=[]  SumI2OutMin=[]  SumI2OutMax=[]  SumI3OutMin=[]  SumI3OutMax=[]  SumDOutMin=[]  SumDOutMax=[]  SaturationOutMin=[]  SaturationOutMax=[]  IntegratorContinuousStateAttributes=''  IntegratorStateMustResolveToSignalObject=off  IntegratorRTWStateStorageClass=Auto  FilterContinuousStateAttributes=''  FilterStateMustResolveToSignalObject=off  FilterRTWStateStorageClass=Auto  DifferentiatorICPrevScaledInput=0  DifferentiatorOutMin=[]  DifferentiatorOutMax=[]
  normalize : Subsystem
  sum : Memory
  Auto Take-off out : Outport
  wires:
  Rotation Pitch/1 -> Rotation pitch switch/1
  Initial Pitch/1 -> Rotation pitch switch/3
  Neutral roll/1 -> Bus Creator/1  "roll"
  Add1/1 -> Thrust_P/1
  Desired Velocity/1 -> Add1/2
  Altitude_P/1 -> Sum1/1
  Add/1 -> Altitude_P/1
  Desired Altitude/1 -> Add/2
  sum/1 -> Sum4/2, Thrust limits/1
  Sum4/1 -> sum/1
  Bus Selector/3 -> Sum5/1  "<heading>"
  Runway direction/1 -> Sum5/2, Bus Creator/6  "yaw"
  Bus Selector/2 -> AltHold pitch switch/2, Altitude Hold/2(Alt), Add/1, Enroute Indicator/2(Altitude)  "<alt>"
  Bus Selector/1 -> Rotation pitch switch/2, Altitude Hold/1(V_ind), Velocity Indicator/1(Velocity), Add1/1  "<V>"
  Sum5/1 -> normalize/1(In)
  normalize/1(Out) -> Yaw_P/1
  Enroute Indicator/1(Indicator) -> Bus Creator/5  "status"
  Bus Creator/1 -> Auto Take-off out/1
  Sensors in/1 -> Bus Selector/1
  AltHold pitch switch/1 -> Bus Creator/2  "pitch"
  Rotation pitch switch/1 -> AltHold pitch switch/3  "pitch"
  Sum1/1 -> Sum4/1
  Thrust_P/1 -> Sum1/2
  AltHold thrust switch/1 -> Bus Creator/3  "thrust"
  Altitude Hold/2(thrust_out) -> AltHold thrust switch/1
  Altitude Hold/1(pitch_out) -> Enroute Indicator/1(pitch control), AltHold pitch switch/1
  Velocity Indicator/1(Indicator) -> AltHold thrust switch/2
  Yaw_P/1 -> NoseWheel limits/1  "noseWheel"
  Thrust limits/1 -> AltHold thrust switch/3
  NoseWheel limits/1 -> Bus Creator/4  "noseWheel"

== system AutonomousControl/Autonomous Controller /Auto enroute ==
  Sensors in : Inport
  WP : Inport  Port=2
  Altitude Hold : Subsystem
  Bus Creator : BusCreator  Inputs='roll','pitch','thrust','yaw','status'
  Bus Selector : BusSelector  OutputSignals=V,lat,lon,alt
  Data Type Conversion : DataTypeConversion  OutDataTypeStr=double
  MATLAB Function2 : MATLAB Function  TreatAsAtomicUnit=on
  Mux : Mux  Inputs=3
  Neutral Roll : Constant  Value=0
  auto Enroute out : Outport
  wires:
  Bus Selector/1 -> Altitude Hold/1(V_ind)  "<V>"
  WP/1 -> MATLAB Function2/2(WP)
  MATLAB Function2/1(targetHeading) -> Bus Creator/4  "yaw"
  MATLAB Function2/2(status) -> Bus Creator/5  "status"
  Neutral Roll/1 -> Bus Creator/1  "roll"
  Bus Creator/1 -> auto Enroute out/1
  Altitude Hold/1(pitch_out) -> Bus Creator/2  "pitch"
  Altitude Hold/2(thrust_out) -> Bus Creator/3  "thrust"
  Sensors in/1 -> Bus Selector/1
  Bus Selector/2 -> Mux/1  "<lat>"
  Bus Selector/3 -> Mux/2  "<lon>"
  Bus Selector/4 -> Altitude Hold/2(Alt), Mux/3  "<alt>"
  Mux/1 -> Data Type Conversion/1
  Data Type Conversion/1 -> MATLAB Function2/1(currentPosition)

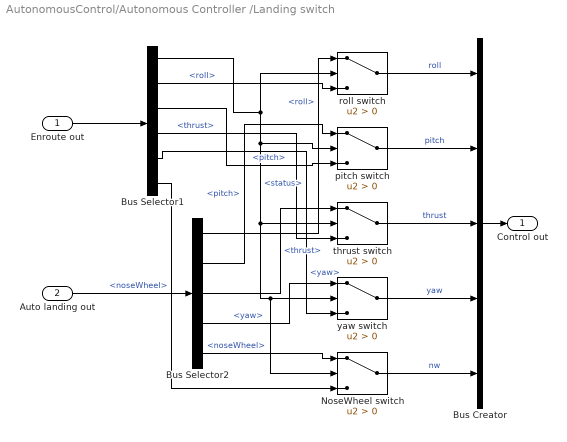
== system AutonomousControl/Autonomous Controller /Landing switch ==
  Enroute out : Inport
  Auto landing out : Inport  Port=2
  Bus Creator : BusCreator  Inputs='roll','pitch','thrust','yaw','nw'
  Bus Selector1 : BusSelector  OutputSignals=status,roll,pitch,thrust,yaw,noseWheel
  Bus Selector2 : BusSelector  OutputSignals=roll,pitch,thrust,yaw,noseWheel
  NoseWheel switch : Switch  Criteria=u2 > Threshold
  pitch switch : Switch  Criteria=u2 > Threshold
  roll switch : Switch  Criteria=u2 > Threshold
  thrust switch : Switch  Criteria=u2 > Threshold
  yaw switch : Switch  Criteria=u2 > Threshold
  Control out : Outport
  wires:
  Bus Selector1/2 -> roll switch/3  "<roll>"
  roll switch/1 -> Bus Creator/1  "roll"
  Bus Selector2/1 -> roll switch/1  "<roll>"
  Bus Selector1/3 -> pitch switch/3  "<pitch>"
  pitch switch/1 -> Bus Creator/2  "pitch"
  Bus Selector2/2 -> pitch switch/1  "<pitch>"
  Bus Selector1/4 -> thrust switch/3  "<thrust>"
  thrust switch/1 -> Bus Creator/3  "thrust"
  Bus Selector2/3 -> thrust switch/1  "<thrust>"
  Bus Selector1/5 -> yaw switch/3  "<yaw>"
  yaw switch/1 -> Bus Creator/4  "yaw"
  Bus Selector2/4 -> yaw switch/1  "<yaw>"
  Bus Selector1/1 -> roll switch/2, NoseWheel switch/2, yaw switch/2, thrust switch/2, pitch switch/2  "<status>"
  Bus Selector1/6 -> NoseWheel switch/3  "<noseWheel>"
  Bus Selector2/5 -> NoseWheel switch/1  "<noseWheel>"
  Enroute out/1 -> Bus Selector1/1
  Auto landing out/1 -> Bus Selector2/1
  Bus Creator/1 -> Control out/1
  NoseWheel switch/1 -> Bus Creator/5  "nw"

== system AutonomousControl/Autonomous Controller /Take-off switch ==
  Auto Take-off out : Inport
  Auto Enroute out : Inport  Port=2
  Bus Creator : BusCreator  Inputs='roll','pitch','thrust','yaw','noseWheel','status'
  Bus Selector : BusSelector  OutputSignals=roll,pitch,thrust,yaw,status
  Bus Selector1 : BusSelector  OutputSignals=status,roll,pitch,thrust,yaw,noseWheel
  pitch switch : Switch  Criteria=u2 > Threshold
  roll switch : Switch  Criteria=u2 > Threshold
  thrust switch : Switch  Criteria=u2 > Threshold
  yaw switch : Switch  Criteria=u2 > Threshold
  Enroute out : Outport
  wires:
  Bus Selector1/2 -> roll switch/3  "<roll>"
  roll switch/1 -> Bus Creator/1  "roll"
  Bus Selector1/3 -> pitch switch/3  "<pitch>"
  pitch switch/1 -> Bus Creator/2  "pitch"
  Bus Selector1/4 -> thrust switch/3  "<thrust>"
  thrust switch/1 -> Bus Creator/3  "thrust"
  Bus Selector1/1 -> yaw switch/2, thrust switch/2, pitch switch/2, roll switch/2  "<status>"
  Bus Selector1/5 -> yaw switch/3  "<yaw>"
  yaw switch/1 -> Bus Creator/4  "yaw"
  Bus Selector/1 -> roll switch/1  "<roll>"
  Bus Selector/2 -> pitch switch/1  "<pitch>"
  Bus Selector/3 -> thrust switch/1  "<thrust>"
  Bus Selector/4 -> yaw switch/1  "<yaw>"
  Auto Enroute out/1 -> Bus Selector/1
  Auto Take-off out/1 -> Bus Selector1/1
  Bus Selector1/6 -> Bus Creator/5  "<noseWheel>"
  Bus Creator/1 -> Enroute out/1
  Bus Selector/5 -> Bus Creator/6  "<status>"

== system AutonomousControl/Get data from XPlane/3-mission time ==
  In2 : Inport
  Memory2 : Memory
  Switch2 : Switch  Criteria=u2 ~= 0
  Out1 : Outport
  wires:
  Memory2/1 -> Switch2/3, Out1/1
  Switch2/1 -> Memory2/1
  In2/1 -> Switch2/1, Switch2/2

== system AutonomousControl/Get data from XPlane/continuous ==
  In2 : Inport
  Memory2 : Memory
  Switch2 : Switch  Criteria=u2 ~= 0
  Out1 : Outport
  wires:
  Memory2/1 -> Switch2/3, Out1/1
  Switch2/1 -> Memory2/1
  In2/1 -> Switch2/1, Switch2/2

== system AutonomousControl/Get data from XPlane/continuous1 ==
  In2 : Inport
  Memory2 : Memory
  Switch2 : Switch  Criteria=u2 ~= 0
  Out1 : Outport
  wires:
  Memory2/1 -> Switch2/3, Out1/1
  Switch2/1 -> Memory2/1
  In2/1 -> Switch2/1, Switch2/2

== system AutonomousControl/Get data from XPlane/continuous10 ==
  In2 : Inport
  Memory2 : Memory
  Switch2 : Switch  Criteria=u2 ~= 0
  Out1 : Outport
  wires:
  Memory2/1 -> Switch2/3, Out1/1
  Switch2/1 -> Memory2/1
  In2/1 -> Switch2/1, Switch2/2

== system AutonomousControl/Get data from XPlane/continuous11 ==
  In2 : Inport
  Memory2 : Memory
  Switch2 : Switch  Criteria=u2 ~= 0
  Out1 : Outport
  wires:
  Memory2/1 -> Switch2/3, Out1/1
  Switch2/1 -> Memory2/1
  In2/1 -> Switch2/1, Switch2/2

== system AutonomousControl/Get data from XPlane/continuous12 ==
  In2 : Inport
  Memory2 : Memory
  Switch2 : Switch  Criteria=u2 ~= 0
  Out1 : Outport
  wires:
  Memory2/1 -> Switch2/3, Out1/1
  Switch2/1 -> Memory2/1
  In2/1 -> Switch2/1, Switch2/2

== system AutonomousControl/Get data from XPlane/continuous13 ==
  In2 : Inport
  Memory2 : Memory
  Switch2 : Switch  Criteria=u2 ~= 0
  Out1 : Outport
  wires:
  Memory2/1 -> Switch2/3, Out1/1
  Switch2/1 -> Memory2/1
  In2/1 -> Switch2/1, Switch2/2

== system AutonomousControl/Get data from XPlane/continuous2 ==
  In2 : Inport
  Memory2 : Memory
  Switch2 : Switch  Criteria=u2 ~= 0
  Out1 : Outport
  wires:
  Memory2/1 -> Switch2/3, Out1/1
  Switch2/1 -> Memory2/1
  In2/1 -> Switch2/1, Switch2/2

== system AutonomousControl/Get data from XPlane/continuous3 ==
  In2 : Inport
  Memory2 : Memory
  Switch2 : Switch  Criteria=u2 ~= 0
  Out1 : Outport
  wires:
  Memory2/1 -> Switch2/3, Out1/1
  Switch2/1 -> Memory2/1
  In2/1 -> Switch2/1, Switch2/2

== system AutonomousControl/Get data from XPlane/continuous4 ==
  In2 : Inport
  Memory2 : Memory
  Switch2 : Switch  Criteria=u2 ~= 0
  Out1 : Outport
  wires:
  Memory2/1 -> Switch2/3, Out1/1
  Switch2/1 -> Memory2/1
  In2/1 -> Switch2/1, Switch2/2

== system AutonomousControl/Get data from XPlane/continuous5 ==
  In2 : Inport
  Memory2 : Memory
  Switch2 : Switch  Criteria=u2 ~= 0
  Out1 : Outport
  wires:
  Memory2/1 -> Switch2/3, Out1/1
  Switch2/1 -> Memory2/1
  In2/1 -> Switch2/1, Switch2/2

== system AutonomousControl/Get data from XPlane/continuous6 ==
  In2 : Inport
  Memory2 : Memory
  Switch2 : Switch  Criteria=u2 ~= 0
  Out1 : Outport
  wires:
  Memory2/1 -> Switch2/3, Out1/1
  Switch2/1 -> Memory2/1
  In2/1 -> Switch2/1, Switch2/2

== system AutonomousControl/Get data from XPlane/continuous7 ==
  In2 : Inport
  Memory2 : Memory
  Switch2 : Switch  Criteria=u2 ~= 0
  Out1 : Outport
  wires:
  Memory2/1 -> Switch2/3, Out1/1
  Switch2/1 -> Memory2/1
  In2/1 -> Switch2/1, Switch2/2

== system AutonomousControl/Get data from XPlane/continuous8 ==
  In2 : Inport
  Memory2 : Memory
  Switch2 : Switch  Criteria=u2 ~= 0
  Out1 : Outport
  wires:
  Memory2/1 -> Switch2/3, Out1/1
  Switch2/1 -> Memory2/1
  In2/1 -> Switch2/1, Switch2/2

== system AutonomousControl/Get data from XPlane/continuous9 ==
  In2 : Inport
  Memory2 : Memory
  Switch2 : Switch  Criteria=u2 ~= 0
  Out1 : Outport
  wires:
  Memory2/1 -> Switch2/3, Out1/1
  Switch2/1 -> Memory2/1
  In2/1 -> Switch2/1, Switch2/2

== system AutonomousControl/Autonomous Controller /Attitude Controller/Yaw deadzone ==
  Roll : Inport
  in : Inport  Port=2
  1-D Lookup Table : Lookup_n-D  NumberOfTableDimensions=1  BreakpointsForDimension1=[0,5,7,10,12.5,15,17,40]  BreakpointsForDimension2=[10,13,17,23,30,40,50]  Table=[1,0.30329,0.16957,0.07655,0.033915,0.010659,0,0]  InternalRulePriority=Speed  RndMeth=Simplest  InputSameDT=on
  Abs : Abs
  Product : Product
  out : Outport
  wires:
  Abs/1 -> 1-D Lookup Table/1
  Roll/1 -> Abs/1
  in/1 -> Product/1
  Product/1 -> out/1
  1-D Lookup Table/1 -> Product/2

== system AutonomousControl/Autonomous Controller /Attitude Controller/normalize ==
  In : Inport
  Minus Offset : Constant  Value=-360
  Offset : Constant  Value=360
  Sum1 : Sum  Inputs=|++
  Sum7 : Sum  Inputs=|++
  Switch : Switch  Criteria=u2 > Threshold  Threshold=-180
  Switch1 : Switch  Criteria=u2 > Threshold  Threshold=180
  Out : Outport
  wires:
  Offset/1 -> Sum7/2
  Sum7/1 -> Switch/3
  In/1 -> Switch/2, Switch/1, Sum1/2, Switch1/2, Sum7/1
  Sum1/1 -> Switch1/1
  Minus Offset/1 -> Sum1/1
  Switch/1 -> Switch1/3
  Switch1/1 -> Out/1

== system AutonomousControl/Autonomous Controller /Auto Landing/Desired Altitude ==
  Alt : Inport
  1-D Lookup Table : Lookup_n-D  NumberOfTableDimensions=1  BreakpointsForDimension1=[5,11,17,23,30,40,50]  Table=[0.6,0.32122,0.14486,0.03905,-0.026066,-0.07219,-0.1]  InternalRulePriority=Speed  RndMeth=Simplest  InputSameDT=on
  pitch : Outport
  wires:
  Alt/1 -> 1-D Lookup Table/1
  1-D Lookup Table/1 -> pitch/1

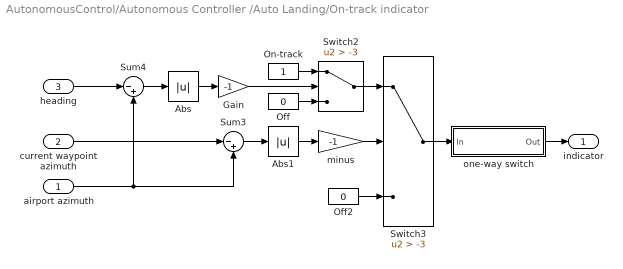
== system AutonomousControl/Autonomous Controller /Auto Landing/On-track indicator ==
  airport azimuth : Inport
  current waypoint azimuth : Inport  Port=2
  heading : Inport  Port=3
  Abs : Abs
  Abs1 : Abs
  Gain : Gain  Gain=-1
  Off : Constant  Value=0
  Off2 : Constant  Value=0
  On-track : Constant
  Sum3 : Sum  Inputs=|-+
  Sum4 : Sum  Inputs=|-+
  Switch2 : Switch  Criteria=u2 > Threshold  Threshold=-3
  Switch3 : Switch  Criteria=u2 > Threshold  Threshold=-3
  minus : Gain  Gain=-1
  "one-way switch " : Subsystem
  indicator : Outport
  wires:
  Sum4/1 -> Abs/1
  On-track/1 -> Switch2/1
  Abs/1 -> Gain/1
  minus/1 -> Switch3/2
  current waypoint azimuth/1 -> Sum3/1
  airport azimuth/1 -> Sum3/2, Sum4/2
  Gain/1 -> Switch2/2
  "one-way switch "/1(Out) -> indicator/1
  Switch3/1 -> "one-way switch "/1(In)
  Off/1 -> Switch2/3
  Switch2/1 -> Switch3/1
  Abs1/1 -> minus/1
  Sum3/1 -> Abs1/1
  Off2/1 -> Switch3/3
  heading/1 -> Sum4/1

== system AutonomousControl/Autonomous Controller /Auto Landing/normalize ==
  In : Inport
  Minus Offset : Constant  Value=-360
  Offset : Constant  Value=360
  Sum1 : Sum  Inputs=|++
  Sum7 : Sum  Inputs=|++
  Switch : Switch  Criteria=u2 > Threshold  Threshold=-180
  Switch1 : Switch  Criteria=u2 > Threshold  Threshold=180
  Out : Outport
  wires:
  Offset/1 -> Sum7/2
  Sum7/1 -> Switch/3
  In/1 -> Switch/2, Switch/1, Sum1/2, Switch1/2, Sum7/1
  Sum1/1 -> Switch1/1
  Minus Offset/1 -> Sum1/1
  Switch/1 -> Switch1/3
  Switch1/1 -> Out/1

== system AutonomousControl/Autonomous Controller /Auto Landing/normalize1 ==
  In : Inport
  Constant : Constant  Value=360
  Sum7 : Sum  Inputs=|++
  Switch : Switch  Criteria=u2 > Threshold  Threshold=-180
  Out : Outport
  wires:
  Switch/1 -> Out/1
  Constant/1 -> Sum7/2
  Sum7/1 -> Switch/3
  In/1 -> Switch/2, Switch/1, Sum7/1

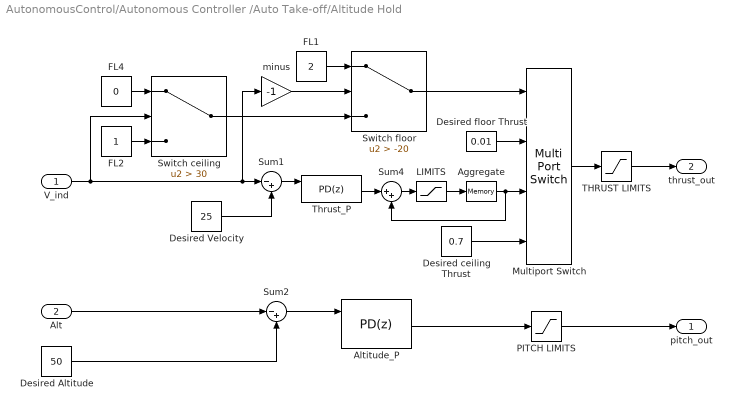
== system AutonomousControl/Autonomous Controller /Auto Take-off/Altitude Hold ==
  V_ind : Inport
  Alt : Inport  Port=2
  Aggregate : Memory
  Altitude_P : simulink/Continuous/PID Controller  Controller=PD  TimeDomain=Discrete-time  SampleTime=0.02  IntegratorMethod=Forward Euler  FilterMethod=Forward Euler  Form=Parallel  UseFilter=off  ControllerParametersSource=internal  P=0.12  I=0.0003  D=0.0024  N=20  InitialConditionSource=internal  InitialConditionForIntegrator=0  InitialConditionForFilter=0  ExternalReset=either  LimitOutput=on  UpperSaturationLimit=1  LowerSaturationLimit=-1  LinearizeAsGain=on  AntiWindupMode=none  Kb=1  TrackingMode=off  Kt=1  PParamMin=[]  PParamMax=[]  IParamMin=[]  IParamMax=[]  DParamMin=[]  DParamMax=[]  NParamMin=[]  NParamMax=[]  KbParamMin=[]  KbParamMax=[]  KtParamMin=[]  KtParamMax=[]  POutMin=[]  POutMax=[]  IOutMin=[]  IOutMax=[]  DOutMin=[]  DOutMax=[]  NOutMin=[]  NOutMax=[]  KbOutMin=[]  KbOutMax=[]  KtOutMin=[]  KtOutMax=[]  IntegratorOutMin=[]  IntegratorOutMax=[]  FilterOutMin=[]  FilterOutMax=[]  SumOutMin=[]  SumOutMax=[]  SumI1OutMin=[]  SumI1OutMax=[]  SumI2OutMin=[]  SumI2OutMax=[]  SumI3OutMin=[]  SumI3OutMax=[]  SumDOutMin=[]  SumDOutMax=[]  SaturationOutMin=[]  SaturationOutMax=[]  IntegratorContinuousStateAttributes=''  IntegratorStateMustResolveToSignalObject=off  IntegratorRTWStateStorageClass=Auto  FilterContinuousStateAttributes=''  FilterStateMustResolveToSignalObject=off  FilterRTWStateStorageClass=Auto  DifferentiatorICPrevScaledInput=0  DifferentiatorOutMin=[]  DifferentiatorOutMax=[]
  Desired Altitude : Constant  Value=50  OutDataTypeStr=single
  Desired Velocity : Constant  Value=25  OutDataTypeStr=single
  "Desired ceiling Thrust " : Constant  Value=0.7  OutDataTypeStr=single
  Desired floor Thrust : Constant  Value=0.01  OutDataTypeStr=single
  FL1 : Constant  Value=2  OutDataTypeStr=single
  FL2 : Constant  OutDataTypeStr=single
  FL4 : Constant  Value=0  OutDataTypeStr=single
  LIMITS : Saturate  UpperLimit=0.4  LowerLimit=0
  Multiport Switch : MultiPortSwitch  DataPortOrder=Zero-based contiguous
  PITCH LIMITS : Saturate  UpperLimit=0.2  LowerLimit=-0.2
  Sum1 : Sum  Inputs=|-+
  Sum2 : Sum  Inputs=|-+
  Sum4 : Sum  Inputs=|++
  Switch ceiling : Switch  Criteria=u2 > Threshold  Threshold=30
  Switch floor : Switch  Criteria=u2 > Threshold  Threshold=-20
  THRUST LIMITS : Saturate  UpperLimit=1  LowerLimit=0
  Thrust_P : simulink/Continuous/PID Controller  Controller=PD  TimeDomain=Discrete-time  SampleTime=0.02  IntegratorMethod=Forward Euler  FilterMethod=Forward Euler  Form=Parallel  UseFilter=off  ControllerParametersSource=internal  P=0.0005  I=0.0000000001  D=0.003  N=20  InitialConditionSource=internal  InitialConditionForIntegrator=0  InitialConditionForFilter=0  ExternalReset=either  LimitOutput=on  UpperSaturationLimit=1  LowerSaturationLimit=-1  LinearizeAsGain=on  AntiWindupMode=none  Kb=1  TrackingMode=off  Kt=1  PParamMin=[]  PParamMax=[]  IParamMin=[]  IParamMax=[]  DParamMin=[]  DParamMax=[]  NParamMin=[]  NParamMax=[]  KbParamMin=[]  KbParamMax=[]  KtParamMin=[]  KtParamMax=[]  POutMin=[]  POutMax=[]  IOutMin=[]  IOutMax=[]  DOutMin=[]  DOutMax=[]  NOutMin=[]  NOutMax=[]  KbOutMin=[]  KbOutMax=[]  KtOutMin=[]  KtOutMax=[]  IntegratorOutMin=[]  IntegratorOutMax=[]  FilterOutMin=[]  FilterOutMax=[]  SumOutMin=[]  SumOutMax=[]  SumI1OutMin=[]  SumI1OutMax=[]  SumI2OutMin=[]  SumI2OutMax=[]  SumI3OutMin=[]  SumI3OutMax=[]  SumDOutMin=[]  SumDOutMax=[]  SaturationOutMin=[]  SaturationOutMax=[]  IntegratorContinuousStateAttributes=''  IntegratorStateMustResolveToSignalObject=off  IntegratorRTWStateStorageClass=Auto  FilterContinuousStateAttributes=''  FilterStateMustResolveToSignalObject=off  FilterRTWStateStorageClass=Auto  DifferentiatorICPrevScaledInput=0  DifferentiatorOutMin=[]  DifferentiatorOutMax=[]
  minus : Gain  Gain=-1
  pitch_out : Outport
  thrust_out : Outport  Port=2
  wires:
  PITCH LIMITS/1 -> pitch_out/1
  Sum2/1 -> Altitude_P/1
  Desired Altitude/1 -> Sum2/2
  Altitude_P/1 -> PITCH LIMITS/1
  Sum1/1 -> Thrust_P/1
  Desired Velocity/1 -> Sum1/2
  Sum4/1 -> LIMITS/1
  Thrust_P/1 -> Sum4/1
  Alt/1 -> Sum2/1
  Switch ceiling/1 -> Switch floor/3
  V_ind/1 -> Switch ceiling/2, minus/1, Sum1/1
  minus/1 -> Switch floor/2
  Switch floor/1 -> Multiport Switch/1
  FL1/1 -> Switch floor/1
  Desired floor Thrust/1 -> Multiport Switch/2
  Multiport Switch/1 -> THRUST LIMITS/1
  FL4/1 -> Switch ceiling/1
  FL2/1 -> Switch ceiling/3
  "Desired ceiling Thrust "/1 -> Multiport Switch/4
  THRUST LIMITS/1 -> thrust_out/1
  LIMITS/1 -> Aggregate/1
  Aggregate/1 -> Multiport Switch/3, Sum4/2

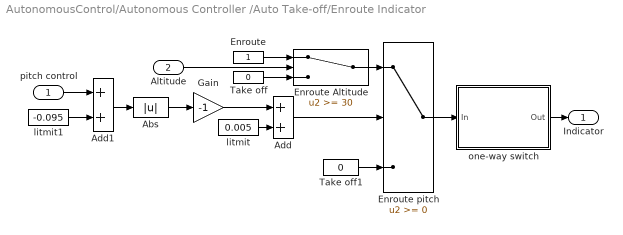
== system AutonomousControl/Autonomous Controller /Auto Take-off/Enroute Indicator ==
  pitch control : Inport
  Altitude : Inport  Port=2
  Abs : Abs
  Add : Sum
  Add1 : Sum
  Enroute : Constant  OutDataTypeStr=single
  Enroute Altitude : Switch  Threshold=30
  Enroute pitch : Switch
  Gain : Gain  Gain=-1
  Take off : Constant  Value=0  OutDataTypeStr=single
  Take off1 : Constant  Value=0  OutDataTypeStr=single
  litmit : Constant  Value=0.005
  litmit1 : Constant  Value=-0.095
  "one-way switch " : Subsystem
  Indicator : Outport
  wires:
  Enroute/1 -> Enroute Altitude/1
  Take off/1 -> Enroute Altitude/3
  Altitude/1 -> Enroute Altitude/2
  "one-way switch "/1(Out) -> Indicator/1
  Abs/1 -> Gain/1
  litmit/1 -> Add/2
  Add/1 -> Enroute pitch/2
  Gain/1 -> Add/1
  Enroute Altitude/1 -> Enroute pitch/1
  Take off1/1 -> Enroute pitch/3
  Enroute pitch/1 -> "one-way switch "/1(In)
  pitch control/1 -> Add1/1
  litmit1/1 -> Add1/2
  Add1/1 -> Abs/1

== system AutonomousControl/Autonomous Controller /Auto Take-off/Velocity Indicator ==
  Velocity : Inport
  Saturated : Constant  OutDataTypeStr=single
  Unsaturated : Constant  Value=0  OutDataTypeStr=single
  "one-way switch " : Subsystem
  switch : Switch  Threshold=25
  Indicator : Outport
  wires:
  Saturated/1 -> switch/1
  Unsaturated/1 -> switch/3
  Velocity/1 -> switch/2
  "one-way switch "/1(Out) -> Indicator/1
  switch/1 -> "one-way switch "/1(In)

== system AutonomousControl/Autonomous Controller /Auto Take-off/normalize ==
  In : Inport
  Minus Offset : Constant  Value=-360
  Offset : Constant  Value=360
  Sum1 : Sum  Inputs=|++
  Sum7 : Sum  Inputs=|++
  Switch : Switch  Criteria=u2 > Threshold  Threshold=-180
  Switch1 : Switch  Criteria=u2 > Threshold  Threshold=180
  Out : Outport
  wires:
  Offset/1 -> Sum7/2
  Sum7/1 -> Switch/3
  In/1 -> Switch/2, Switch/1, Sum1/2, Switch1/2, Sum7/1
  Sum1/1 -> Switch1/1
  Minus Offset/1 -> Sum1/1
  Switch/1 -> Switch1/3
  Switch1/1 -> Out/1
